simulink model "exemplo1sim_caso2"  (R2024a)
settings: Solver=VariableStepAuto  StartTime=0.0  StopTime=10.0  RelTol=1e-3
values from neighbouring files (symbols this model uses):
  A = [-3, 0; 0, -2]    [exemplo1.m]    (also in exemplo1_Caso2.m; exemplo1_Caso3.m)
  B = [1; 1]    [exemplo1.m]    (also in exemplo1_Caso2.m; exemplo1_Caso3.m)
  C = [1, 2]    [exemplo1.m]    (also in exemplo1_Caso2.m; exemplo1_Caso3.m)
  ci_x1 = 0.4    [exemplo1.m]    (also in exemplo1_Caso2.m; exemplo1_Caso3.m)
  ci_x2 = 0.2    [exemplo1.m]    (also in exemplo1_Caso2.m; exemplo1_Caso3.m)
  Ke = K'    [exemplo1.m]    (also in exemplo1_Caso2.m; exemplo1_Caso3.m)
  sys = ss(A, B, C, D)    [exemplo1.m]    (also in exemplo1_Caso2.m; exemplo1_Caso3.m)
libraries: simulink x1
settings Model: Creator=caugu  LastModifiedBy=caugu

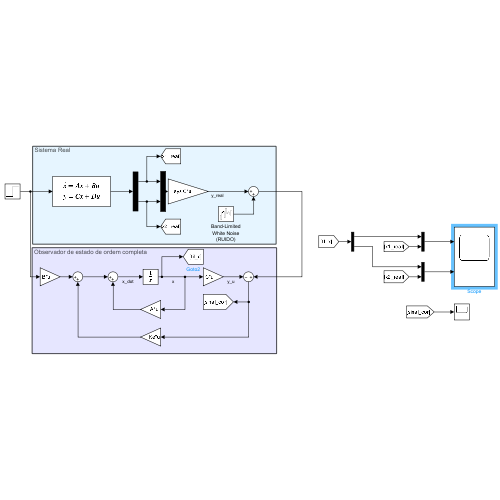
[thumbnail: Simulink's stored preview of the top-level diagram]
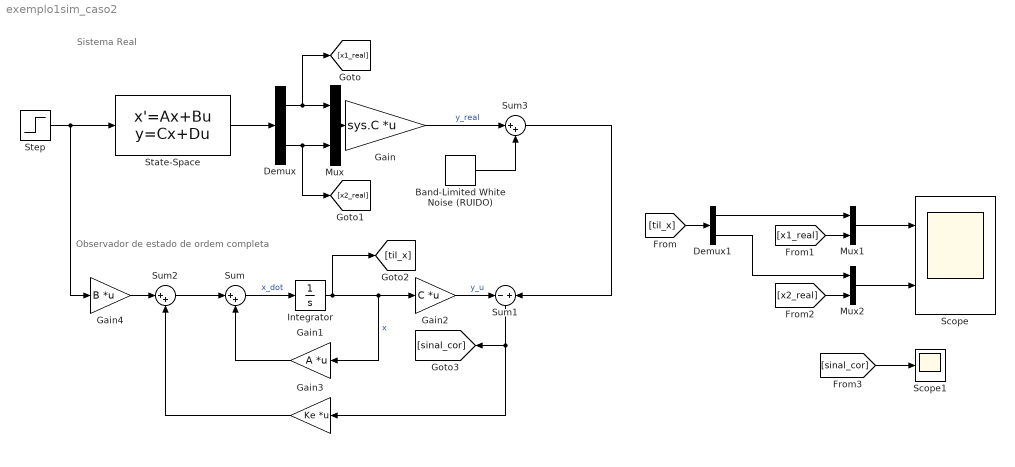
== system exemplo1sim_caso2 ==
  note: Sistema Real
  note: Observador de estado de ordem completa
  Band-Limited White Noise (RUIDO) : simulink/Sources/Band-Limited White Noise  Cov=[1e-4]  Ts=0.1  seed=[23341]
  Demux : Demux  Outputs=2
  Demux1 : Demux  Outputs=2
  Gain : Gain  Gain=sys.C  Multiplication=Matrix(K*u)
  Gain1 : Gain  Gain=A  Multiplication=Matrix(K*u)
  Gain2 : Gain  Gain=C  Multiplication=Matrix(K*u)
  Gain3 : Gain  Gain=Ke  Multiplication=Matrix(K*u)
  Gain4 : Gain  Gain=B  Multiplication=Matrix(K*u)
  Integrator : Integrator  InitialCondition=[ci_x1; ci_x2]
  Mux : Mux  Inputs=2
  Mux1 : Mux  Inputs=2
  Mux2 : Mux  Inputs=2
  Scope : Scope  NumInputPorts=2
  Scope1 : Scope
  State-Space : StateSpace  A=sys.A  B=sys.B  C=eye(2)  D=zeros(2,1)  InitialCondition=0
  Step : Step  Time=0  SampleTime=0
  Sum : Sum  Inputs=|++
  Sum1 : Sum  Inputs=-+
  Sum2 : Sum  Inputs=|++
  Sum3 : Sum  Inputs=|++
  wires:
  State-Space/1 -> Demux/1
  Demux/1 -> [x1_real], Mux/1
  Demux/2 -> [x2_real], Mux/2
  Step/1 -> Gain4/1, State-Space/1
  Mux/1 -> Gain/1
  Sum/1 -> Integrator/1  "x_dot"
  Integrator/1 -> [til_x], Gain2/1, Gain1/1  "x"
  Gain1/1 -> Sum/2
  Gain2/1 -> Sum1/1  "y_u"
  Sum1/1 -> Gain3/1, [sinal_cor]
  Sum2/1 -> Sum/1
  Gain4/1 -> Sum2/1
  Gain3/1 -> Sum2/2
  [til_x] -> Demux1/1
  Demux1/1 -> Mux1/1
  [x1_real] -> Mux1/2
  Demux1/2 -> Mux2/1
  [x2_real] -> Mux2/2
  Mux1/1 -> Scope/1
  Mux2/1 -> Scope/2
  [sinal_cor] -> Scope1/1
  Sum3/1 -> Sum1/2
  Gain/1 -> Sum3/1  "y_real"
  Band-Limited White Noise (RUIDO)/1 -> Sum3/2
